simulink model "ftm_three_phase_pwm_s32k11x"  (Simulink 9.0)
settings: Solver=FixedStepDiscrete  StartTime=0.0  StopTime=10.0  FixedStep=1  RelTol=1e-3
InitFcn:
  | mbd_s32k_consistency_checks(bdroot(gcs));
undefined symbols (not defined in the file): LQFP, thumb
libraries: mbd_s32k1xx_ec_toolbox x15, simulink x1
Description:
  | This sample shows how to use FTM modules to generate PWM signals for the S32K118 MCUs three phase PWM.
  | The model generates  PWM in the Combine mode on Ch0/Ch1, Ch2/Ch3 and Ch4/Ch5 outputs of the FTM0 module,
  | a channel interrupt on Ch0 and a fault interrupt when the active state of the pin PA7 is High. The PWM also can be
  | enabled and disabled when needs be. Also, the duty cycle, (set and clear points for each pair), frequency and deadtime
  | can be changed using the ftm_three_phase_pwm_output_s32k11x.pmp FreeMaster example.
  | 
  | Validation:
  | Connect pin J1.4   (PTE0) with the pin J1.14 (PTD3/SW3) on S32K118
  | Connect pin J2.6   (PTB2)  to the scope to watch FTM0 channel 0 output
  | Connect pin J2.5   (PTB3)  to the scope to watch FTM0 channel 1 output
  | Connect pin J4.7   (PTC14) to the scope to watch FTM0 channel 2 output
  | Connect pin J4.9   (PTC15) to the scope to watch FTM0 channel 3 output
  | Connect pin J1.5   (PTA12) to the scope to watch FTM0 channel 6 output
  | Connect pin J1.7   (PTA13) to the scope to watch FTM0 channel 7 output
  | 
  | Each channel output frequency should be 10kHz, and the deadband between each PWM signals for each pair of channels
  | should be 500nsec just like in the attatched graphs (Ch0/Ch1).
  | The first two pairs are set Active High - Main inverted.
  | The last PWM pair is set Active High - Main duplicated.
  | 
  | The RGB LED lights green, because of the CH ISR Handler.
  | When the SW3 is pressed, the Fault Handler lights the RGB LED red, and the PWM signals are stopped.
  | The SW2 enables and disables the PWM Module and toggles the blue led.
settings Model: Creator=NXP MBDT Team  LastModifiedBy=nxf35172
settings DataIOCC: ExternalInput=off  InitialState=off  SaveFormat=Dataset  SaveOutput=off  SignalLogging=off  SaveTime=off
settings OptimizationCC: DefaultParameterBehavior=Inlined  PassReuseOutputArgsAs=Individual arguments  LifeSpan=auto
settings DebuggingCC: UnderspecifiedInitializationDetection=Simplified  MergeDetectMultiDrivingBlocksExec=error  InheritedTsInSrcMsg=none  SingleTaskRateTransMsg=error  ParameterTunabilityLossMsg=error  UnconnectedInputMsg=error  UnconnectedOutputMsg=error  UnconnectedLineMsg=error  UnknownTsInhSupMsg=error  SFUnexpectedBacktrackingDiag=error  SFNoUnconditionalDefaultTransitionDiag=error  SFExecutionAtInitializationDiag=warning
settings HardwareCC: ProdLargestAtomicInteger=Long  ProdLargestAtomicFloat=Double  ProdIntDivRoundTo=Zero  ProdEndianess=LittleEndian  ProdHWDeviceType=ARM Compatible->ARM Cortex
settings ModelReferenceCC: PropagateSignalLabelsOutOfModel=on
settings SFSimCC: MATLABDynamicMemAlloc=off
settings RTWCC: SystemTargetFile=mbd_s32k.tlc  MakeCommand=mbd_s32k_make_rtw COPY_MDLREF_INCLUDES=0  TemplateMakefile=mbd_s32k.tmf  Description=Model Based Design Toolbox S32K14x Code Generation Target  GenerateReport=on  IncludeHyperlinkInReport=on  LaunchReport=on  GenerateTraceInfo=on  GenerateTraceReport=on  GenerateTraceReportSl=on  GenerateTraceReportSf=on  GenerateTraceReportEml=on
settings CodeAppCC: ForceParamTrailComments=on  IgnoreCustomStorageClasses=off  OperatorAnnotations=on  SimulinkDataObjDesc=on  SFDataObjDesc=on  InsertBlockDesc=on  StateflowObjectComments=off
settings STFCustomTargetCC: TargetLangStandard=C99 (ISO)  MultiwordLength=256  CombineOutputUpdateFcns=on  ERTCustomFileBanners=on  SupportContinuousTime=off  SupportNonInlinedSFcns=off  RemoveResetFunc=on  MATLABClassNameForMDSCustomization=Simulink.SoftwareTarget.ERTCustomization  GRTInterface=off  SystemTargetFile=mbd_s32k.tlc
settings ERTTargetCC: TargetLangStandard=C99 (ISO)  ParMdlRefBuildCompliant=off  CompOptLevelCompliant=off  ConcurrentExecutionCompliant=off  ModelStepFunctionPrototypeControlCompliant=off  CPPClassGenCompliant=off  UseToolchainInfoCompliant=off  InlinedParameterPlacement=NonHierarchical  ERTSrcFileBannerTemplate=mbd_ert_code_template.cgt  ERTHdrFileBannerTemplate=mbd_ert_code_template.cgt  ERTDataSrcFileTemplate=mbd_ert_code_template.cgt  ERTDataHdrFileTemplate=mbd_ert_code_template.cgt  ERTCustomFileTemplate=example_file_process.tlc
settings ConfigComp: CovMetricSettings=dwe  CovHtmlReporting=off  CovSaveCumulativeToWorkspaceVar=off  CovSaveSingleToWorkspaceVar=off  CovExternalEMLEnable=on

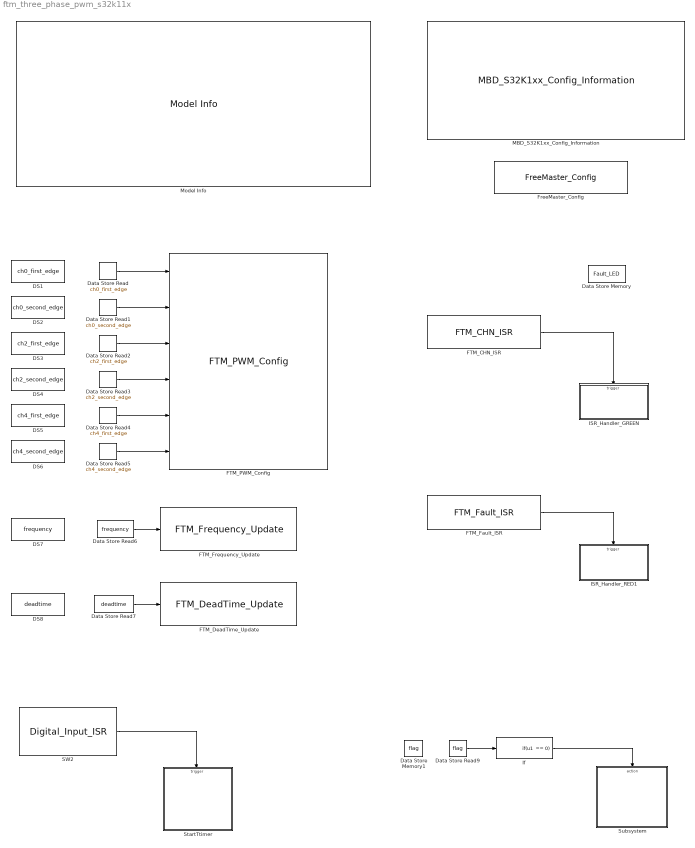
== system ftm_three_phase_pwm_s32k11x ==
  DS1 : DataStoreMemory  DataStoreName=ch0_first_edge  ReadBeforeWriteMsg=warning  WriteAfterWriteMsg=warning  WriteAfterReadMsg=warning  ShowAdditionalParam=off  OutDataTypeStr=single
  DS2 : DataStoreMemory  DataStoreName=ch0_second_edge  ReadBeforeWriteMsg=warning  WriteAfterWriteMsg=warning  WriteAfterReadMsg=warning  InitialValue=0.8  ShowAdditionalParam=off  OutDataTypeStr=single
  DS3 : DataStoreMemory  DataStoreName=ch2_first_edge  ReadBeforeWriteMsg=warning  WriteAfterWriteMsg=warning  WriteAfterReadMsg=warning  ShowAdditionalParam=off  OutDataTypeStr=single
  DS4 : DataStoreMemory  DataStoreName=ch2_second_edge  ReadBeforeWriteMsg=warning  WriteAfterWriteMsg=warning  WriteAfterReadMsg=warning  InitialValue=0.5  ShowAdditionalParam=off  OutDataTypeStr=single
  DS5 : DataStoreMemory  DataStoreName=ch4_first_edge  ReadBeforeWriteMsg=warning  WriteAfterWriteMsg=warning  WriteAfterReadMsg=warning  InitialValue=0.5  ShowAdditionalParam=off  OutDataTypeStr=single
  DS6 : DataStoreMemory  DataStoreName=ch4_second_edge  ReadBeforeWriteMsg=warning  WriteAfterWriteMsg=warning  WriteAfterReadMsg=warning  InitialValue=0.75  ShowAdditionalParam=off  OutDataTypeStr=single
  DS7 : DataStoreMemory  DataStoreName=frequency  ReadBeforeWriteMsg=warning  WriteAfterWriteMsg=warning  WriteAfterReadMsg=warning  InitialValue=10000  ShowAdditionalParam=off  OutDataTypeStr=uint32
  DS8 : DataStoreMemory  DataStoreName=deadtime  ReadBeforeWriteMsg=warning  WriteAfterWriteMsg=warning  WriteAfterReadMsg=warning  InitialValue=500  ShowAdditionalParam=off  OutDataTypeStr=uint32
  Data Store Memory : DataStoreMemory  DataStoreName=Fault_LED  ReadBeforeWriteMsg=warning  WriteAfterWriteMsg=warning  WriteAfterReadMsg=warning  ShowAdditionalParam=off  OutDataTypeStr=boolean
  Data Store Memory1 : DataStoreMemory  DataStoreName=flag  ReadBeforeWriteMsg=warning  WriteAfterWriteMsg=warning  WriteAfterReadMsg=warning  ShowAdditionalParam=off
  Data Store Read : DataStoreRead  DataStoreName=ch0_first_edge
  Data Store Read1 : DataStoreRead  DataStoreName=ch0_second_edge
  Data Store Read2 : DataStoreRead  DataStoreName=ch2_first_edge
  Data Store Read3 : DataStoreRead  DataStoreName=ch2_second_edge
  Data Store Read4 : DataStoreRead  DataStoreName=ch4_first_edge
  Data Store Read5 : DataStoreRead  DataStoreName=ch4_second_edge
  Data Store Read6 : DataStoreRead  DataStoreName=frequency
  Data Store Read7 : DataStoreRead  DataStoreName=deadtime
  Data Store Read9 : DataStoreRead  DataStoreName=flag
  FTM_CHN_ISR : mbd_s32k1xx_ec_toolbox/Motor Control Blocks/FTM Blocks/FTM_CHN_ISR  Priority=10  ftmModule=1  channel=0  isrlevel=0  mcuTargetUpdate=on
  FTM_DeadTime_Update : mbd_s32k1xx_ec_toolbox/Motor Control Blocks/FTM Blocks/FTM_DeadTime_Update  Priority=10  ftmModule=1  mcuTargetUpdate=on  deadtimeUnits=Nanoseconds  deadtimePrescaler=Divide by 1
  FTM_Fault_ISR : mbd_s32k1xx_ec_toolbox/Motor Control Blocks/FTM Blocks/FTM_Fault_ISR  Priority=10  ftmModule=1  faultChannel=2  isrPriority=15  mcuTargetUpdate=on
  FTM_Frequency_Update : mbd_s32k1xx_ec_toolbox/Motor Control Blocks/FTM Blocks/FTM_Frequency_Update  Priority=10  ftmModule=1  mcuTargetUpdate=on  ftmPwmUnits=Hz
  FTM_PWM_Config : mbd_s32k1xx_ec_toolbox/Motor Control Blocks/FTM Blocks/FTM_PWM_Config  Priority=1  ftmModule=1  ftmMode=Combine mode PWM  ftmSourceClock=40 MHz  swcontrol_enable=off  chan0En=on  chan0Type=Independent  chan2En=on  chan2Type=Independent  chan4En=off  chan4Type=Independent  chan6En=on  chan6Type=Independent  ftmPwmUnits=Hz  outFrequency=10000  ftmPeriod=4000  ftmPrescaler=Divide by 1  deadtimeUnits=Nanoseconds  deadtimeNs=100  deadtimeTicks=4  deadtimePrescaler=Divide by 1  dutyCycleCh0=0.25  dutyCycleCh1=0.25  dutyCycleCh2=0.25  dutyCycleCh3=0.25  dutyCycleCh4=0.25  dutyCycleCh5=0.25  dutyCycleCh6=0.25  dutyCycleCh7=0.25  dutyCycleSim=off  startAfterInit=on  showAdvOpt=on  pinFtmCh0=PTB2: [FTM1_CH0 | FTM Channel]  pinFtmCh1=PTB3: [FTM1_CH1 | FTM Channel]  pinPolCh0=Active High  pinPolCh1=Active Low  outputComplem0=Main inverted  outputLevel0=Low  outputLevel1=Low  pinFtmCh2=PTC14: [FTM1_CH2 | FTM Channel]  pinFtmCh3=PTC15: [FTM1_CH3 | FTM Channel]  pinPolCh2=Active High  pinPolCh3=Active Low  outputComplem2=Main inverted  outputLevel2=Low  outputLevel3=Low  pinFtmCh4=PTA10: [FTM1_CH4 | FTM Channel]  pinFtmCh5=PTA11: [FTM1_CH5 | FTM Channel]  pinPolCh4=Active High  pinPolCh5=Active Low  outputComplem4=Main inverted  outputLevel4=Low  outputLevel5=Low  pinFtmCh6=PTA12: [FTM1_CH6 | FTM Channel]  pinFtmCh7=PTA13: [FTM1_CH7 | FTM Channel]  pinPolCh6=Active High  pinPolCh7=Active Low  outputComplem6=Main duplicated  outputLevel6=Low  outputLevel7=Low  initTrigger=off  chTrigger0=on  chTrigger1=off  chTrigger2=off  chTrigger3=off  chTrigger4=off  chTrigger5=off  chTrigger6=off  chTrigger7=off  mcuTargetUpdate=on  pwmSyncTrg=Software trigger  pwmSyncHwRouting=TRGMUX_FTM7  pwmSyncTrg0=off  pwmSyncTrg1=off  pwmSyncTrg2=off  pwmSyncAutoClear=on  pwmSyncMinLoad=on  pwmSyncMaxLoad=on  pwmSyncInvert=System Clock  pwmSyncOutControl=System Clock  pwmSyncOutMask=System Clock  pwmSyncCounterInitial=System Clock  pwmSyncPoints=Update now  reloadEnable=off  reloadPriority=0  reloadHalfCycle=off  reloadHCR=0  reloadFrequency=0  chnMatch0=off  chnMatch1=off  chnMatch2=off  chnMatch3=off  chnMatch4=off  chnMatch5=off  chnMatch6=off  chnMatch7=off  pwmFaultProtection=on  pwmFaultInterrupt=on  pwmFaultClearing=Automatic Fault control for all channels  pwmFaultPinState=Safe Value  pwmFaultFilterValue=0  pwmFaultPriority=1  fault_disen_0=off  fault_filter_0=off  fault_polarity_0=Active High  fault_disen_1=off  fault_filter_1=off  fault_polarity_1=Active high  fault_disen_2=on  fault_filter_2=off  fault_polarity_2=Active high  fault_disen_3=off  fault_filter_3=off  fault_polarity_3=Active high  fault_pin_0=None  fault_pin_1=None  fault_pin_2=PTE0: [FTM1_FLT2 | FTM Fault Input]  fault_pin_3=None
  FreeMaster_Config : mbd_s32k1xx_ec_toolbox/Utility Blocks/FreeMaster_Config  interface=LPUART0  baudrate=115200  rxd=PTB0: [LPUART0_RX | Receive]  txd=PTB1: [LPUART0_TX | Transmit]  mode=Short Interrupt  isr_prio=0  show_adv_opts=on  use_scope=on  max_scope_vars=8  use_recorder=on  max_rec_vars=8  rec_buff_size=1024  rec_timebase=0 seconds  comm_buffer_size_auto=on  comm_buffer_size=255  comm_rqueue_size_default=on  comm_rqueue_size=32
  ISR_Handler_GREEN : Subsystem
  ISR_Handler_RED1 : Subsystem
  If : If  IfExpression="u1  == 0"  ShowElse=off
  MBD_S32K1xx_Config_Information : mbd_s32k1xx_ec_toolbox/MBD_S32K1xx_Config_Information  mbdt_ver=0  disp_str=|  config_params=[]  mcu_target_name=S32K118  mcu_target_package=64-LQFP  mcu_target_sram_size=25KB  mcu_system_clock_freq=40  mcu_xtal_freq=External 40  mcu_steptick_timer=LPIT Channel 0  mcu_steptick_prio=3  ds_import_enable=on  target_compiler=GCC  target_memory=FLASH  gcc_target_compile_opts=-mcpu=cortex-m0plus -mthumb -O1 -g -gstrict-dwarf  gcc_target_assemble_opts=-mcpu=cortex-m0plus -mthumb -g  gcc_target_link_opts=-mcpu=cortex-m0plus -mthumb  gcc_target_default_lcf=on  gcc_target_user_lcf=S32K118_25_flash.ld  ghs_target_compile_opts=-mcpu=cortexm0plus -mthumb -fsoft -Ogeneral -Wundef -Wimplicit-int -Wshadow -Wtrigraphs --no_commons --gnu_asm -gnu99 -gdwarf-2 -G  ghs_target_assemble_opts=-mcpu=cortexm0plus -mthumb -fsoft --gnu_asm  ghs_target_link_opts=-mcpu=cortexm0plus -mthumb -fsoft  ghs_target_default_lcf=on  ghs_target_user_lcf=S32K118_25_flash.ld  iar_target_compile_opts=--thumb -Ol -e --debug --dlib_config normal  iar_target_assemble_opts=--thumb  iar_target_link_opts=--no_exceptions --vfe --inline  iar_target_default_lcf=on  iar_target_user_lcf=S32K118_25_flash.icf  pil_download_enable=off  rbl_download_enable=on  rbl_start_delay=5000  rbl_download_interface=OpenSDA  rbl_restart_request=off  rbl_com_port=Custom  rbl_com_port_custom=COM1  pil_download_rate=57600  pil_opensda_drive=Custom  pil_opensda_drive_custom=D  pil_uart_instance=0  pil_uart_rx=PTA2: [LPUART0_RX | Receive]  pil_uart_tx=PTA3: [LPUART0_TX | Transmit]  FTM_PWM_PcrCheckEnDis=on  FTM_Input_Edge_Inputs_PcrCheckEnDis=on  FTM_Dual_Edge_Inputs_PcrCheckEnDis=on  FTM_Quadrature_Inputs_PcrCheckEnDis=on  FTM_Hall_Sensor_Inputs_PcrCheckEnDis=on  LPTMR_PcrCheckEnDis=on  PIT_PcrCheckEnDis=on  RTC_PcrCheckEnDis=on  FlexCAN_PcrCheckEnDis=on  LIN_PcrCheckEnDis=on  FlexIO_PcrCheckEnDis=on  LPI2C_PcrCheckEnDis=on  LPSPI_PcrCheckEnDis=on  LPUART_PcrCheckEnDis=on  CMP_PcrCheckEnDis=on  GPIO_OutputPcrCheckEnDis=on  GPIO_InputPcrCheckEnDis=on  SBC_PcrCheckEnDis=on  AMMCLIB_PcrCheckEnDis=on  FM_PcrCheckEnDis=on  Profile_PcrCheckEnDis=on  ConfigParams_PcrCheckEnDis=on  ModelRef_PcrCheckEnDis=on  PDB0_PcrCheckEnDis=on  CSEc_PcrCheckEnDis=on  eDMA_PcrCheckEnDis=on  ADC_PcrCheckEnDis=on  WDOG_PcrCheckEnDis=on
      | Target : S32K144-64KB_SRAM
      | Package : 100-pin
      | System clock : 80 MHz
      | XTAL clock : External 8 MHz
      | Compiler : IAR
      | Target Type : FLASH
      | Download Code after build : off
      | Step Tick Interrupt Priority : 15
  Model Info : simulink/Model-Wide Utilities/Model Info  Frame=off  DisplayStringWithTags=|  HorizontalTextAlignment=Left  LeftAlignmentValue=0.02
      | Model Name: %<ModelName>
      | 
      | Description: %<Description>
  SW2 : mbd_s32k1xx_ec_toolbox/GPIO Blocks/Digital_Input_ISR  gpio_pin=PTD5: [PTD5 | Port D I/O]  irqc=on rising-edge  prio=3
  StartTtimer : Subsystem
  Subsystem : Subsystem
  wires:
  Data Store Read/1 -> FTM_PWM_Config/1
  Data Store Read3/1 -> FTM_PWM_Config/4
  Data Store Read4/1 -> FTM_PWM_Config/5
  Data Store Read5/1 -> FTM_PWM_Config/6
  Data Store Read2/1 -> FTM_PWM_Config/3
  Data Store Read1/1 -> FTM_PWM_Config/2
  Data Store Read6/1 -> FTM_Frequency_Update/1
  Data Store Read7/1 -> FTM_DeadTime_Update/1
  FTM_Fault_ISR/1 -> ISR_Handler_RED1/Trigger
  FTM_CHN_ISR/1 -> ISR_Handler_GREEN/Trigger
  Data Store Read9/1 -> If/1
  If/1 -> Subsystem/Action
  SW2/1 -> StartTtimer/Trigger

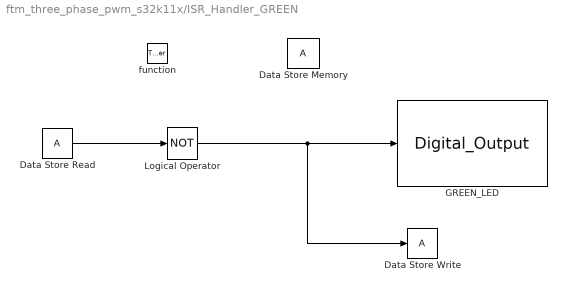
== system ftm_three_phase_pwm_s32k11x/ISR_Handler_GREEN ==
  function : TriggerPort  TriggerType=function-call  VariantControl=Variant
  Data Store Memory : DataStoreMemory  ReadBeforeWriteMsg=warning  WriteAfterWriteMsg=warning  WriteAfterReadMsg=warning  ShowAdditionalParam=off  OutDataTypeStr=boolean
  Data Store Read : DataStoreRead
  Data Store Write : DataStoreWrite
  GREEN_LED : mbd_s32k1xx_ec_toolbox/GPIO Blocks/Digital_Output  gpio_pin=PTD16: [PTD16 | Port D I/O]  init_val=Low  drive_strength=High
  Logical Operator : Logic  Operator=NOT  AllPortsSameDT=off  OutDataTypeStr=boolean
  wires:
  Data Store Read/1 -> Logical Operator/1
  Logical Operator/1 -> Data Store Write/1, GREEN_LED/1

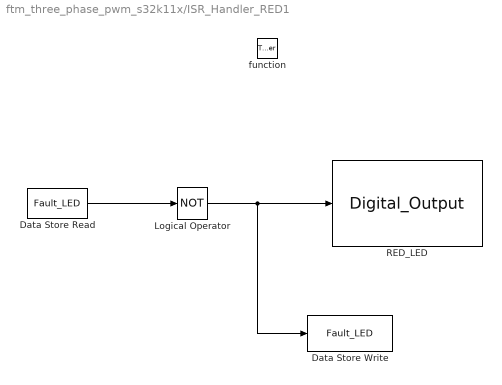
== system ftm_three_phase_pwm_s32k11x/ISR_Handler_RED1 ==
  function : TriggerPort  TriggerType=function-call  VariantControl=Variant
  Data Store Read : DataStoreRead  DataStoreName=Fault_LED
  Data Store Write : DataStoreWrite  DataStoreName=Fault_LED
  Logical Operator : Logic  Operator=NOT  AllPortsSameDT=off  OutDataTypeStr=boolean
  RED_LED : mbd_s32k1xx_ec_toolbox/GPIO Blocks/Digital_Output  gpio_pin=PTD15: [PTD15 | Port D I/O]  init_val=Low  drive_strength=High
  wires:
  Logical Operator/1 -> Data Store Write/1, RED_LED/1
  Data Store Read/1 -> Logical Operator/1

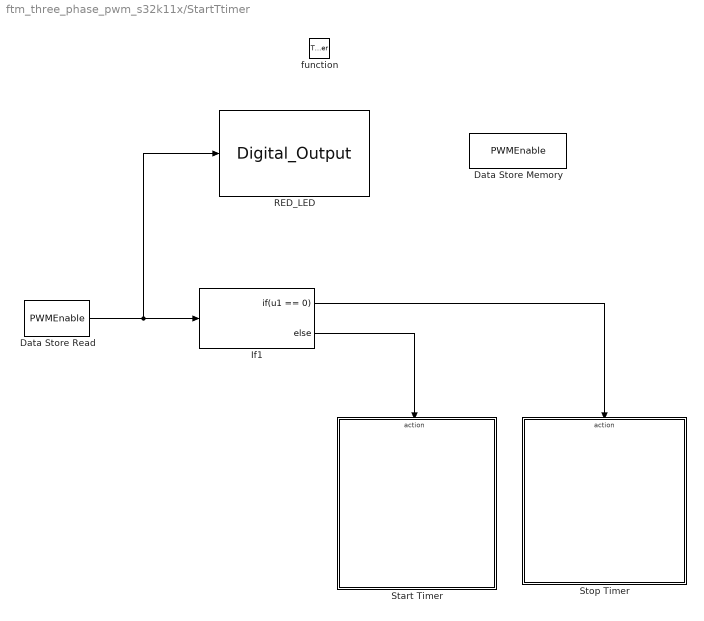
== system ftm_three_phase_pwm_s32k11x/StartTtimer ==
  function : TriggerPort  TriggerType=function-call  VariantControl=Variant
  Data Store Memory : DataStoreMemory  DataStoreName=PWMEnable  ReadBeforeWriteMsg=warning  WriteAfterWriteMsg=warning  WriteAfterReadMsg=warning  ShowAdditionalParam=off  OutDataTypeStr=boolean
  Data Store Read : DataStoreRead  DataStoreName=PWMEnable
  If1 : If  IfExpression=u1 == 0
  RED_LED : mbd_s32k1xx_ec_toolbox/GPIO Blocks/Digital_Output  gpio_pin=PTE8: [PTE8 | Port E I/O]  init_val=Low  drive_strength=High
  Start Timer : Subsystem
  Stop Timer : Subsystem
  wires:
  Data Store Read/1 -> RED_LED/1, If1/1
  If1/2 -> Start Timer/Action
  If1/1 -> Stop Timer/Action

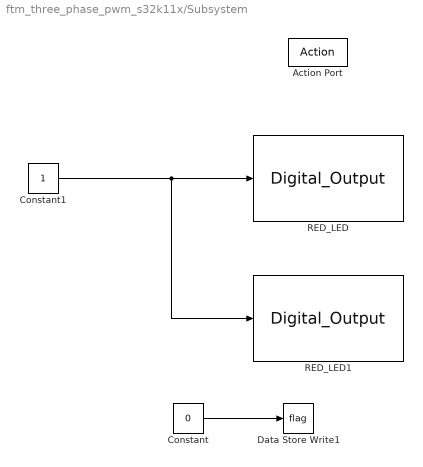
== system ftm_three_phase_pwm_s32k11x/Subsystem ==
  Action Port : ActionPort
  Constant : Constant  Value=0
  Constant1 : Constant  OutDataTypeStr=boolean
  Data Store Write1 : DataStoreWrite  DataStoreName=flag
  RED_LED : mbd_s32k1xx_ec_toolbox/GPIO Blocks/Digital_Output  gpio_pin=PTD15: [PTD15 | Port D I/O]  init_val=Low  drive_strength=High
  RED_LED1 : mbd_s32k1xx_ec_toolbox/GPIO Blocks/Digital_Output  gpio_pin=PTE8: [PTE8 | Port E I/O]  init_val=Low  drive_strength=High
  wires:
  Constant/1 -> Data Store Write1/1
  Constant1/1 -> RED_LED1/1, RED_LED/1

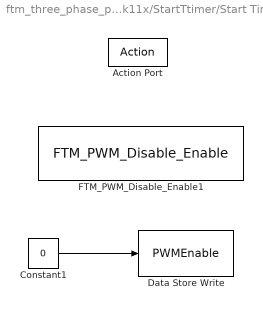
== system ftm_three_phase_pwm_s32k11x/StartTtimer/Start Timer ==
  Action Port : ActionPort
  Constant1 : Constant  Value=0  OutDataTypeStr=boolean
  Data Store Write : DataStoreWrite  DataStoreName=PWMEnable
  FTM_PWM_Disable_Enable1 : mbd_s32k1xx_ec_toolbox/Motor Control Blocks/FTM Blocks/FTM_PWM_Disable_Enable  Priority=1  ftmModule=1  action=Enable
  wires:
  Constant1/1 -> Data Store Write/1

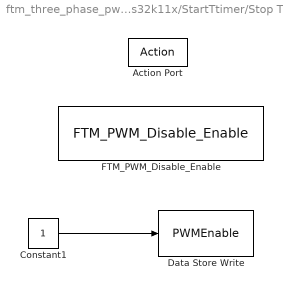
== system ftm_three_phase_pwm_s32k11x/StartTtimer/Stop Timer ==
  Action Port : ActionPort
  Constant1 : Constant  OutDataTypeStr=boolean
  Data Store Write : DataStoreWrite  DataStoreName=PWMEnable
  FTM_PWM_Disable_Enable : mbd_s32k1xx_ec_toolbox/Motor Control Blocks/FTM Blocks/FTM_PWM_Disable_Enable  Priority=1  ftmModule=1  action=Disable
  wires:
  Constant1/1 -> Data Store Write/1
